simulink model "MultirotorSim"  (R2020b)
settings: Solver=VariableStepAuto  StartTime=0.0  StopTime=Simulation.T_END  MaxStep=Simulation.TS_MAX  RelTol=1e-3  EnableMultiTasking=on
PreLoadFcn:
  | InitializeParametersQuadcopterAIAAv3;
undefined symbols (not defined in the file or in its folder): Initial, Uav
settings Model: Creator=jban039  LastModifiedBy=jeremie
settings DataIOCC: Decimation=10
settings OptimizationCC: LifeSpan=inf
settings DebuggingCC: UnconnectedLineMsg=none  AllowSymbolicDim=off  SFUnexpectedBacktrackingDiag=warning  SFNoUnconditionalDefaultTransitionDiag=warning  SFExecutionAtInitializationDiag=none  ArithmeticOperatorsInVariantConditions=warning
settings ModelReferenceCC: ModelReferenceMinAlgLoopOccurrences=on  PropagateSignalLabelsOutOfModel=off
settings SFSimCC: SimUseLocalCustomCode=off  CustomCodeUndefinedFunction=UseInterfaceOnly
settings RTWCC: RTWUseLocalCustomCode=off
settings CodeAppCC: StateflowObjectComments=on
settings GRTTargetCC: TargetLangStandard=C89/C90 (ANSI)
settings ConfigComp: CovMetricSettings=dw  CovSaveCumulativeToWorkspaceVar=on  CovSaveSingleToWorkspaceVar=on  CovExternalEMLEnable=off

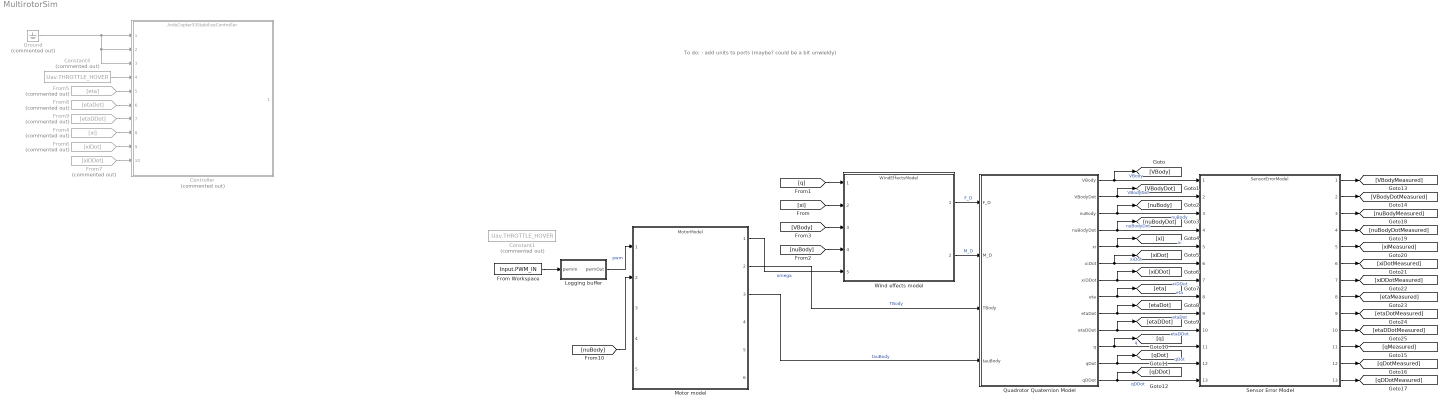
== system MultirotorSim ==
  note: To do:
      |
      | - add units  to ports (maybe? could be a bit unwieldy)
  Constant1 : Constant  Commented=on  Value=Uav.THROTTLE_HOVER
  Constant4 : Constant  Commented=on  Value=Uav.THROTTLE_HOVER
  Controller : ModelReference  Commented=on  ModelNameDialog=ArduCopter33StabilizeController  SimulationMode=Normal  ModelReferenceVersion=1.9
  From Workspace : FromWorkspace  VariableName=Input.PWM_IN
  From4 : From  Commented=on  GotoTag=xi
  From5 : From  Commented=on  GotoTag=eta
  From6 : From  Commented=on  GotoTag=xiDot
  From7 : From  Commented=on  GotoTag=xiDDot
  From8 : From  Commented=on  GotoTag=etaDot
  From9 : From  Commented=on  GotoTag=etaDDot
  Ground : Ground  Commented=on
  Logging buffer : Subsystem
  Motor model : ModelReference  ModelNameDialog=MotorModel  SimulationMode=Normal  ModelReferenceVersion=5.0
  Quadrotor Quaternion Model : Subsystem
  Sensor Error Model : ModelReference  ModelNameDialog=SensorErrorModel  SimulationMode=Normal  ModelReferenceVersion=5.0
  Wind effects model : ModelReference  ModelNameDialog=WindEffectsModel  SimulationMode=Normal  ModelReferenceVersion=1.65
  wires:
  Motor model/1 -> Wind effects model/5  "omega"
  Motor model/2 -> Quadrotor Quaternion Model/3(TBody)  "TBody"
  Motor model/3 -> Quadrotor Quaternion Model/4(tauBody)  "tauBody"
  Wind effects model/2 -> Quadrotor Quaternion Model/2(M_D)  "M_D"
  Quadrotor Quaternion Model/1(VBody) -> Sensor Error Model/1, [VBody]  "VBody"
  Quadrotor Quaternion Model/2(VBodyDot) -> Sensor Error Model/2, [VBodyDot]  "VBodyDot"
  Quadrotor Quaternion Model/3(nuBody) -> [nuBody], Sensor Error Model/3  "nuBody"
  Quadrotor Quaternion Model/4(nuBodyDot) -> Sensor Error Model/4, [nuBodyDot]  "nuBodyDot"
  Quadrotor Quaternion Model/5(xi) -> Sensor Error Model/5, [xi]  "xi"
  Quadrotor Quaternion Model/6(xiDot) -> Sensor Error Model/6, [xiDot]  "xiDot"
  Quadrotor Quaternion Model/7(xiDDot) -> Sensor Error Model/7, [xiDDot]  "xiDDot"
  Quadrotor Quaternion Model/8(eta) -> Sensor Error Model/8, [eta]  "eta"
  Quadrotor Quaternion Model/9(etaDot) -> Sensor Error Model/9, [etaDot]  "etaDot"
  Quadrotor Quaternion Model/10(etaDDot) -> [etaDDot], Sensor Error Model/10  "etaDDot"
  [q] -> Wind effects model/1
  [xi] -> Wind effects model/2
  [nuBody] -> Wind effects model/4
  [VBody] -> Wind effects model/3
  From5/1 -> Controller/5
  From4/1 -> Controller/8
  From6/1 -> Controller/9
  From7/1 -> Controller/10
  From8/1 -> Controller/6
  From9/1 -> Controller/7
  Ground/1 -> Controller/3, Controller/2, Controller/1
  Constant4/1 -> Controller/4
  [nuBody] -> Motor model/2
  From Workspace/1 -> Logging buffer/1(pwmIn)
  Quadrotor Quaternion Model/11(q) -> Sensor Error Model/11, [q]  "q"
  Quadrotor Quaternion Model/12(qDot) -> [qDot], Sensor Error Model/12  "qDot"
  Quadrotor Quaternion Model/13(qDDot) -> Sensor Error Model/13, [qDDot]  "qDDot"
  Wind effects model/1 -> Quadrotor Quaternion Model/1(F_D)  "F_D"
  Sensor Error Model/1 -> [VBodyMeasured]
  Sensor Error Model/2 -> [VBodyDotMeasured]
  Sensor Error Model/3 -> [nuBodyMeasured]
  Sensor Error Model/4 -> [nuBodyDotMeasured]
  Sensor Error Model/5 -> [xiMeasured]
  Sensor Error Model/6 -> [xiDotMeasured]
  Sensor Error Model/7 -> [xiDDotMeasured]
  Sensor Error Model/8 -> [etaMeasured]
  Sensor Error Model/9 -> [etaDotMeasured]
  Sensor Error Model/10 -> [etaDDotMeasured]
  Sensor Error Model/11 -> [qMeasured]
  Sensor Error Model/12 -> [qDotMeasured]
  Sensor Error Model/13 -> [qDDotMeasured]
  Logging buffer/1(pwmOut) -> Motor model/1  "pwm"

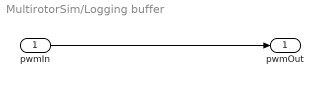
== system MultirotorSim/Logging buffer ==
  pwmIn : Inport
  pwmOut : Outport  VectorParamsAs1DForOutWhenUnconnected=off
  wires:
  pwmIn/1 -> pwmOut/1

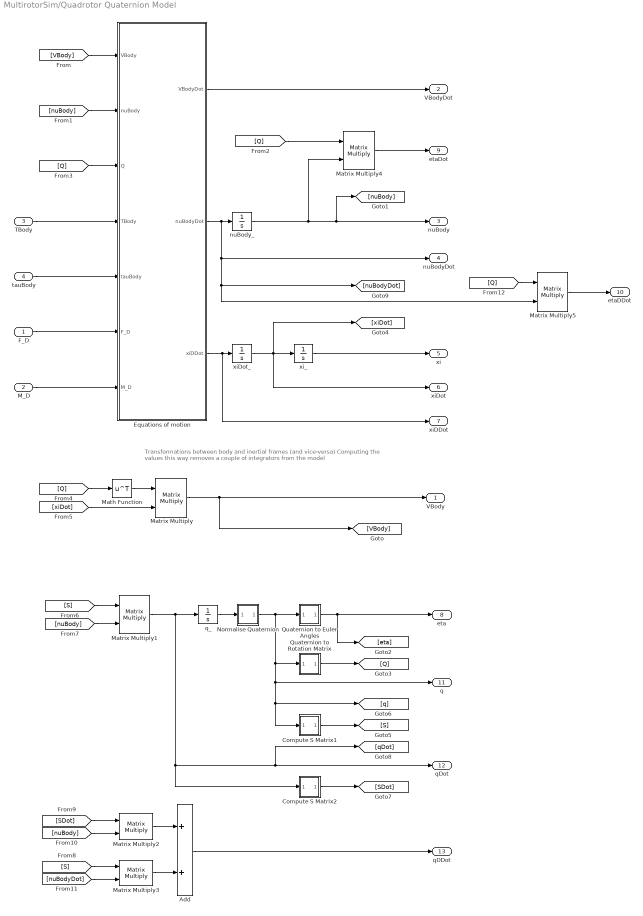
== system MultirotorSim/Quadrotor Quaternion Model ==
  note: Transformations between body and inertial frames (and vice-versa)
      | Computing the values this way removes a couple of integrators from the model
  F_D : Inport
  M_D : Inport  Port=2
  TBody : Inport  Port=3
  tauBody : Inport  Port=4
  Add : Sum
  Compute S Matrix1 : Subsystem  AncestorBlock=QuaternionLibrary/Compute S Matrix
      mask help: Convert an orientation quaternion to an orthogonal transformation matrix
      mask Help:
      | Convert a quaternion
      | [q1 q2 q3 q4]
      | to the S matrix used to compute angular acceleration and velocity quaternion
      | qDot = S * nuBody
      | 
      | qDDot = SDot * nuBody + S * nuBodyDot
      mask Display: disp('S')
  Compute S Matrix2 : Subsystem  AncestorBlock=QuaternionLibrary/Compute S Matrix
      mask help: Convert an orientation quaternion to an orthogonal transformation matrix
      mask Help:
      | Convert a quaternion
      | [q1 q2 q3 q4]
      | to the S matrix used to compute angular acceleration and velocity quaternion
      | qDot = S * nuBody
      | 
      | qDDot = SDot * nuBody + S * nuBodyDot
      mask Display: disp('S')
  Equations of motion : MATLAB Function  TreatAsAtomicUnit=on
  Math Function : Math  Operator=transpose  SignedPower=on  SaturateOnIntegerOverflow=on
  Matrix Multiply{,1..5} (6 alike) : Product  Multiplication=Matrix(*)
  Normalise Quaternion : Subsystem  AncestorBlock=QuaternionLibrary/Normalise Quaternion
      mask help:
      | Normalise a quaternion
      |
      | Qhat = Q / |Q|
      mask Display: disp('Q/|Q|')
  Quaternion to Euler Angles : Subsystem  AncestorBlock=QuaternionLibrary/Quaternion to Euler Angles
      mask help: Convert an orientation quaternion to a vector of Euler angles
      mask Help:
      | Convert an orientation quaternion
      | [q1 q2 q3 q4]
      | where:
      | - q1 is the rotation in radians
      | - [q2 q3 q4] is the vector around which the rotation is performed)
      | to a vector of Euler angles
      | [roll, pitch, yaw]
      | Based on code from the PX4 firmware: https://github.com/PX4/Firmware
      mask Display: disp('Q2E')
  Quaternion to Rotation Matrix : Subsystem  AncestorBlock=QuaternionLibrary/Quaternion to Rotation Matrix
      mask help: Convert an orientation quaternion to an orthogonal transformation matrix
      mask Help:
      | Convert an orientation quaternion
      | [q1 q2 q3 q4]
      | where:
      | - q1 is the rotation in radians
      | - [q2 q3 q4] is the vector around which the rotation is performed)
      | to an orthogonal transformation matrix
      | Based on code from the PX4 firmware: https://github.com/PX4/Firmware
      mask Display: disp('Q2R')
  nuBody_ : Integrator  InitialCondition=Initial.NU_BODY
  q_ : Integrator  InitialCondition=Initial.Q
  xiDot_ : Integrator  InitialCondition=Initial.XI_DOT
  xi_ : Integrator  InitialCondition=Initial.XI
  VBody : Outport  VectorParamsAs1DForOutWhenUnconnected=off
  VBodyDot : Outport  Port=2  VectorParamsAs1DForOutWhenUnconnected=off
  nuBody : Outport  Port=3  VectorParamsAs1DForOutWhenUnconnected=off
  nuBodyDot : Outport  Port=4  VectorParamsAs1DForOutWhenUnconnected=off
  xi : Outport  Port=5  VectorParamsAs1DForOutWhenUnconnected=off
  xiDot : Outport  Port=6  VectorParamsAs1DForOutWhenUnconnected=off
  xiDDot : Outport  Port=7  VectorParamsAs1DForOutWhenUnconnected=off
  eta : Outport  Port=8  VectorParamsAs1DForOutWhenUnconnected=off
  etaDot : Outport  Port=9  VectorParamsAs1DForOutWhenUnconnected=off
  etaDDot : Outport  Port=10  VectorParamsAs1DForOutWhenUnconnected=off
  q : Outport  Port=11  VectorParamsAs1DForOutWhenUnconnected=off
  qDot : Outport  Port=12  VectorParamsAs1DForOutWhenUnconnected=off
  qDDot : Outport  Port=13  VectorParamsAs1DForOutWhenUnconnected=off
  wires:
  Equations of motion/1(VBodyDot) -> VBodyDot/1
  xiDot_/1 -> xi_/1, [xiDot], xiDot/1
  xi_/1 -> xi/1
  [nuBody] -> Equations of motion/2(nuBody)
  [VBody] -> Equations of motion/1(VBody)
  tauBody/1 -> Equations of motion/5(tauBody)
  TBody/1 -> Equations of motion/4(TBody)
  Equations of motion/3(xiDDot) -> xiDot_/1, xiDDot/1
  F_D/1 -> Equations of motion/6(F_D)
  Matrix Multiply/1 -> VBody/1, [VBody]
  M_D/1 -> Equations of motion/7(M_D)
  nuBody_/1 -> Matrix Multiply4/2, [nuBody], nuBody/1
  Equations of motion/2(nuBodyDot) -> nuBody_/1, nuBodyDot/1, Matrix Multiply5/2, [nuBodyDot]
  q_/1 -> Normalise Quaternion/1(quaternion)
  Quaternion to Euler Angles/1(euler) -> eta/1, [eta]
  Matrix Multiply4/1 -> etaDot/1
  Quaternion to Rotation Matrix/1(rotationMatrix) -> [Q]
  [Q] -> Equations of motion/3(Q)
  [Q] -> Math Function/1
  [xiDot] -> Matrix Multiply/2
  Math Function/1 -> Matrix Multiply/1
  [S] -> Matrix Multiply1/1
  [nuBody] -> Matrix Multiply1/2
  Compute S Matrix2/1(rotationMatrix) -> [SDot]
  [S] -> Matrix Multiply3/1
  Matrix Multiply1/1 -> qDot/1, [qDot], Compute S Matrix2/1(quaternion), q_/1
  [SDot] -> Matrix Multiply2/1
  [nuBody] -> Matrix Multiply2/2
  [nuBodyDot] -> Matrix Multiply3/2
  Matrix Multiply2/1 -> Add/1
  Matrix Multiply3/1 -> Add/2
  Normalise Quaternion/1(normalised) -> Quaternion to Euler Angles/1(quaternion), q/1, Compute S Matrix1/1(quaternion), [q], Quaternion to Rotation Matrix/1(quaternion)
  Compute S Matrix1/1(rotationMatrix) -> [S]
  [Q] -> Matrix Multiply4/1
  Add/1 -> qDDot/1
  [Q] -> Matrix Multiply5/1
  Matrix Multiply5/1 -> etaDDot/1

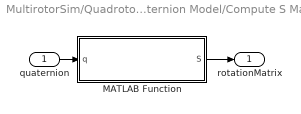
== system MultirotorSim/Quadrotor Quaternion Model/Compute S Matrix1 ==
  quaternion : Inport
  MATLAB Function : MATLAB Function  TreatAsAtomicUnit=on
  rotationMatrix : Outport  VectorParamsAs1DForOutWhenUnconnected=off
  wires:
  quaternion/1 -> MATLAB Function/1(q)
  MATLAB Function/1(S) -> rotationMatrix/1

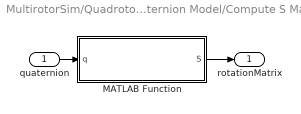
== system MultirotorSim/Quadrotor Quaternion Model/Compute S Matrix2 ==
  quaternion : Inport
  MATLAB Function : MATLAB Function  TreatAsAtomicUnit=on
  rotationMatrix : Outport  VectorParamsAs1DForOutWhenUnconnected=off
  wires:
  quaternion/1 -> MATLAB Function/1(q)
  MATLAB Function/1(S) -> rotationMatrix/1

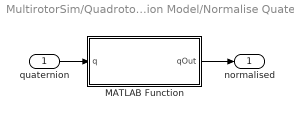
== system MultirotorSim/Quadrotor Quaternion Model/Normalise Quaternion ==
  quaternion : Inport
  MATLAB Function : MATLAB Function  TreatAsAtomicUnit=on
  normalised : Outport  VectorParamsAs1DForOutWhenUnconnected=off
  wires:
  quaternion/1 -> MATLAB Function/1(q)
  MATLAB Function/1(qOut) -> normalised/1

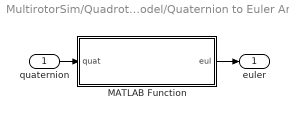
== system MultirotorSim/Quadrotor Quaternion Model/Quaternion to Euler Angles ==
  quaternion : Inport
  MATLAB Function : MATLAB Function  TreatAsAtomicUnit=on
  euler : Outport  VectorParamsAs1DForOutWhenUnconnected=off
  wires:
  quaternion/1 -> MATLAB Function/1(quat)
  MATLAB Function/1(eul) -> euler/1

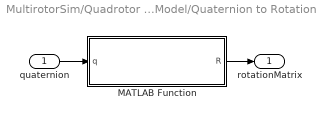
== system MultirotorSim/Quadrotor Quaternion Model/Quaternion to Rotation Matrix ==
  quaternion : Inport
  MATLAB Function : MATLAB Function  TreatAsAtomicUnit=on
  rotationMatrix : Outport  VectorParamsAs1DForOutWhenUnconnected=off
  wires:
  MATLAB Function/1(R) -> rotationMatrix/1
  quaternion/1 -> MATLAB Function/1(q)

== matlab function MultirotorSim/Quadrotor Quaternion Model/Equations of motion ==
  data: VBody input; VBodyDot output; nuBody input; Q input; TBody input size=3; tauBody input size=3; F_D input size=3; M_D input size=3; nuBodyDot output; Uav parameter; xiDDot output
function [VBodyDot, nuBodyDot, xiDDot] = QuadrotorQuaternionModel(...
    VBody, nuBody, Q, TBody, tauBody, F_D, M_D, Uav)
%#codegen

%% Rotation matrices

%% Moments and Forces
% Body frame accelerations
VBodyDot  = (1/Uav.M) * (Q'*Uav.G + TBody - cross(nuBody, Uav.M*VBody) - F_D);
nuBodyDot = Uav.I \ (tauBody - cross(nuBody, Uav.I*nuBody) - M_D);

% Inertial frame accelerations
xiDDot = (1/Uav.M)*(Uav.G + Q*(TBody - F_D));
% etaDDot = WInvertDot*nuBody + WInvert*nuBodyDot;

% Check centripetal force in inertial frame
% F_C = R*cross(nuBody,m*VBody);
end

== matlab function MultirotorSim/Quadrotor Quaternion Model/Quaternion to Rotation Matrix/MATLAB Function ==
  data: q input; R output
function R = QuatToRot( q )
%QUATTOROT Convert quaternion to rotation matrix
%   Written by:    J.X.J. Bannwarth, 2017/03/27
%   Last modified: J.X.J. Bannwarth, 2018/12/11
    W = q(1);
    X = q(2);
    Y = q(3);
    Z = q(4);
    
    xx = X * X;
    xy = X * Y;
    xz = X * Z;
    xw = X * W;

    yy = Y * Y;
    yz = Y * Z;
    yw = Y * W;
    
    zz = Z * Z;
    zw = Z * W;

    m00 = 1 - 2 * ( yy + zz );
    m01 =     2 * ( xy - zw );
    m02 =     2 * ( xz + yw );

    m10 =     2 * ( xy + zw );
    m11 = 1 - 2 * ( xx + zz );
    m12 =     2 * ( yz - xw );

    m20 =     2 * ( xz - yw );
    m21 =     2 * ( yz + xw );
    m22 = 1 - 2 * ( xx + yy );
    
    R = [m00 m01 m02;
         m10 m11 m12;
         m20 m21 m22];   
end

== matlab function MultirotorSim/Quadrotor Quaternion Model/Quaternion to Euler Angles/MATLAB Function ==
  data: quat input; eul output
function eul   = QuaternionToEuler( quat )
%QUATERNIONTOEULER Convert quaternion to euler angles
%   Based on PX4 Firmware code: https://github.com/PX4/Firmware
%   Written by:    J.X.J. Bannwarth, 2016/08/29
%   Last modified: J.X.J. Bannwarth, 2018/12/11

    eul = [ atan2(2.0 .* (quat(1) .* quat(2) + quat(3) .* quat(4)), ...
                1.0 - 2.0 .* (quat(2) .* quat(2) + quat(3) .* quat(3)));
	        asin(2.0 .* (quat(1) .* quat(3) - quat(4) .* quat(2)));
            atan2(2.0 .* (quat(1) .* quat(4) + quat(2) .* quat(3)), ...
                1.0 - 2.0 .* (quat(3) .* quat(3) + quat(4) .* quat(4))) ];
end

== matlab function MultirotorSim/Quadrotor Quaternion Model/Compute S Matrix2/MATLAB Function ==
  data: q input; S output
function S = ComputeSMatrix(q)
%COMPUTESMATRIX Compute S Matrix
%   Written by:    J.X.J. Bannwarth, 2017/03/28
%   Last modified: J.X.J. Bannwarth, 2018/12/11
    S = zeros( 4, 3 );
    S(1,1) = -q(2) * 0.5;
    S(1,2) = -q(3) * 0.5;
    S(1,3) = -q(4) * 0.5;
    S(2,1) =  q(1) * 0.5;
    S(2,2) = -q(4) * 0.5;
    S(2,3) =  q(3) * 0.5;
    S(3,1) =  q(4) * 0.5;
    S(3,2) =  q(1) * 0.5;
    S(3,3) = -q(2) * 0.5;
    S(4,1) = -q(3) * 0.5;
    S(4,2) =  q(2) * 0.5;
    S(4,3) =  q(1) * 0.5;
end

== matlab function MultirotorSim/Quadrotor Quaternion Model/Normalise Quaternion/MATLAB Function ==
  data: q input; qOut output
function qOut = NormaliseQuat( q )
%NORMALISEQUAT Normalise quaternion
%   Based on PX4 Firmware code: https://github.com/PX4/Firmware
%   Written by:    J.X.J. Bannwarth, 2018/12/11
%   Last modified: J.X.J. Bannwarth, 2018/12/11

    qOut = zeros(4,1);
    normVal = sqrt( dot( q, q ) );
    if normVal ~= 0
        qOut = q ./ normVal;
    end
end

== matlab function MultirotorSim/Quadrotor Quaternion Model/Compute S Matrix1/MATLAB Function ==
  data: q input; S output
function S = ComputeSMatrix(q)
%COMPUTESMATRIX Compute S Matrix
%   Written by:    J.X.J. Bannwarth, 2017/03/28
%   Last modified: J.X.J. Bannwarth, 2018/12/11
    S = zeros( 4, 3 );
    S(1,1) = -q(2) * 0.5;
    S(1,2) = -q(3) * 0.5;
    S(1,3) = -q(4) * 0.5;
    S(2,1) =  q(1) * 0.5;
    S(2,2) = -q(4) * 0.5;
    S(2,3) =  q(3) * 0.5;
    S(3,1) =  q(4) * 0.5;
    S(3,2) =  q(1) * 0.5;
    S(3,3) = -q(2) * 0.5;
    S(4,1) = -q(3) * 0.5;
    S(4,2) =  q(2) * 0.5;
    S(4,3) =  q(1) * 0.5;
end
